simulink model "ex11impefk"  (R2025b)
settings: Solver=ode4  StartTime=0.0  StopTime=60  FixedStep=0.05  RelTol=1e-3
settings Model: Creator=Esteban  LastModifiedBy=Esteban

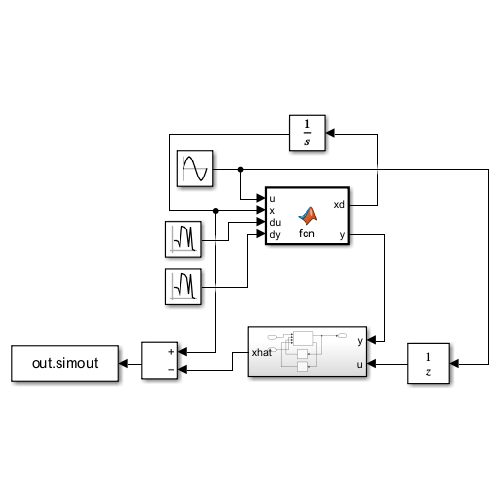
[thumbnail: Simulink's stored preview of the top-level diagram]
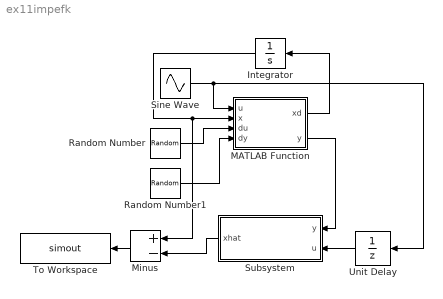
== system ex11impefk ==
  Integrator : Integrator  InitialCondition=[-7/2;4]
  MATLAB Function : MATLAB Function  TreatAsAtomicUnit=on
  Minus : Sum  Inputs=+-
  Random Number : RandomNumber  Variance=0.01  SampleTime=0.05
  Random Number1 : RandomNumber  Variance=0.01  SampleTime=0.05
  Sine Wave : Sin  Amplitude=1.1  Frequency=1.5  SampleTime=0
  Subsystem : Subsystem
  To Workspace : ToWorkspace  VariableName=simout  SaveFormat=Timeseries  SampleTime=-1
  Unit Delay : UnitDelay  SampleTime=-1  HasFrameUpgradeWarning=on
  wires:
  Random Number/1 -> MATLAB Function/3(du)
  Random Number1/1 -> MATLAB Function/4(dy)
  MATLAB Function/1(xd) -> Integrator/1
  Integrator/1 -> Minus/1, MATLAB Function/2(x)
  Sine Wave/1 -> Unit Delay/1, MATLAB Function/1(u)
  MATLAB Function/2(y) -> Subsystem/1(y)
  Unit Delay/1 -> Subsystem/2(u)
  Subsystem/1(xhat) -> Minus/2
  Minus/1 -> To Workspace/1

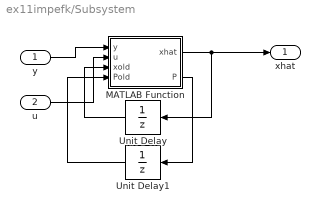
== system ex11impefk/Subsystem ==
  y : Inport
  u : Inport  Port=2
  MATLAB Function : MATLAB Function  TreatAsAtomicUnit=on
  Unit Delay : UnitDelay  InitialCondition=[0;0]  SampleTime=-1  HasFrameUpgradeWarning=on
  Unit Delay1 : UnitDelay  InitialCondition=zeros(2)  SampleTime=-1  HasFrameUpgradeWarning=on
  xhat : Outport
  wires:
  y/1 -> MATLAB Function/1(y)
  u/1 -> MATLAB Function/2(u)
  MATLAB Function/1(xhat) -> Unit Delay/1, xhat/1
  MATLAB Function/2(P) -> Unit Delay1/1
  Unit Delay/1 -> MATLAB Function/3(xold)
  Unit Delay1/1 -> MATLAB Function/4(Pold)

== matlab function ex11impefk/Subsystem/MATLAB Function ==
  data: y input; u input; xhat output; xold input; Pold input; P output
function [xhat,P] = fcn(y,u,xold,Pold)

tau = 0.1;
Qd = eye(2);
Rd = 20;

f=[xold(2);
    -6/5*xold(1)^3+xold(1)-u-3*xold(2)];
J = [0 1
    -18/5*xold(1)^2+1 -3];

F = eye(2) + tau*J;

xp = xold + tau*f;
Pp = F*Pold*F' + Qd;

H = [1 0];

S = H*Pp*H' + Rd;

K = Pp*H' / S;

agg = y-H*xp;

xhat = xp + K*agg;
P = (eye(2)-K*H)*Pp;

== matlab function ex11impefk/MATLAB Function ==
  data: xd output; u input; y output; x input; du input; dy input
function [xd,y] = fcn(u,x,du,dy)

xd=[x(2);
    -6/5*x(1)^3+x(1)-u-3*x(2)+du];
y = x(1)+dy;
